simulink model "RoboBoatVU_2014_Athena"  (R2014a)
settings: Solver=FixedStepDiscrete  StartTime=0.0  StopTime=inf  FixedStep=.1  RelTol=1e-3
undefined symbols (not defined in the file): Com1, Com2, Com3, Com4, DiscIntNeverNeededParam, RGB24, standard, strel
libraries: visiontextngfix x25, dspmtrx3 x22, simulink x19, xpcseriallib x12, slrtlib x7, speedgoatlib_IO102 x6, dspstat3 x5, visionstatistics x3, dspindex x2, xpcvideousblib x2, xpcvideoutillib x2, visionmorphops x1
(part 2 of 4)

== matlab function RoboBoatVU_2014_Athena/Main FSM/Start Speed Gate/Start Speed Gate - Color/Nav Finished ==
  data: Timer input; Finished output; Timeout input; EndGPS input; Latitude input; Longitude input
function Finished = NavFinished(Timer, Timeout, EndGPS, Latitude, Longitude)

%Written by Anderson Lebbad on August 23, 2013
%Last Edited by:

%Checks the timeout and GPS location to determine if the navigation block
%is done. If either one is flagged, the finished signal is sent.


%Parse input GPS and convert angles to radians
CurLat = (floor(Latitude/100)+mod(Latitude,100)/60)*pi/180;
CurLong = (floor(Longitude/100)+mod(Longitude,100)/60)*pi/180;
DesLat = (floor(EndGPS(1)/100)+mod(EndGPS(1),100)/60)*pi/180;
DesLong = (floor(EndGPS(2)/100)+mod(EndGPS(2),100)/60)*pi/180;


%Initialize output
Finished = 0;


%Difference between lats and longs
DiffLat = DesLat - CurLat;
DiffLong = DesLong - CurLong;


%Radius of the earth in meters
R = 6378137;


%Calculate distance using the great-circle distance formula
%Formula documented here:
%   http://www.movable-type.co.uk/scripts/latlong.html
a = sin(DiffLat/2)^2+sin(DiffLong/2)^2*cos(CurLat)*cos(DesLat);
c = 2*atan2(sqrt(a), sqrt(1-a));
Distance = R*c;


%Check timeout and distance, minimum distance to pass a finished signal is
%set to 2 meters
if (Timer > Timeout) || (Distance < 2)
    Finished = 1;
end

== matlab function RoboBoatVU_2014_Athena/Parameters/Task Selector/Message Composer2 ==
  data: taskStrInit input; taskStrAdj output
function taskStrAdj = composeMessage(taskStrInit)
%Written by Anderson Lebbad on August 9, 2013
%Last Edited: Edward Zhu on June 2, 2014

%This function adjusts the length of a vector to a set value by filling
%the remaining space with 0's. This is necessary for data store objects
%that have a fixed size for the memory allocation, but a variable length
%input.

%Length of message packet
strLength = 8;

%Size of text in message
taskStrLength = size(taskStrInit,1);

%Pad end of text with zeros
taskStrAdj = [taskStrInit' zeros(1,strLength-taskStrLength)];

== matlab function RoboBoatVU_2014_Athena/Parameters/Task Selector/Message Composer5 ==
  data: taskStrInit input; taskStrAdj output
function taskStrAdj = composeMessage(taskStrInit)
%Written by Anderson Lebbad on August 9, 2013
%Last Edited: Edward Zhu on June 2, 2014

%This function adjusts the length of a vector to a set value by filling
%the remaining space with 0's. This is necessary for data store objects
%that have a fixed size for the memory allocation, but a variable length
%input.

%Length of message packet
strLength = 8;

%Size of text in message
taskStrLength = size(taskStrInit,1);

%Pad end of text with zeros
taskStrAdj = [taskStrInit' zeros(1,strLength-taskStrLength)];

== matlab function RoboBoatVU_2014_Athena/Main FSM/Start Speed Gate/Start Speed Gate - Color/Buoy Decisions/Nav Logic ==
  data: Compass input; RedBBox input; GreenBBox input; RedCentroid input; GreenCentroid input; Course input; RedDist output; GreenDist output; RPM output; DesiredHeading output; Timer input
function [RedDist, GreenDist, RPM, DesiredHeading] = NavLogic(Compass,...
    RedBBox, GreenBBox, RedCentroid, GreenCentroid, Course, Timer)

%Written by Anderson Lebbad on August 20, 2013
%Last Edited by:

%Determines the signals for driving through the buoy channel based on the
%bounding box and centroid signals from both the red and green detection
%blocks.


%Initialize Outputs
RPM = 2800;
DesiredHeading = Compass;



%% First, calculate the distance each detected polyform A-0 buoy is.

%The buoy has a fixed diameter (m), the camera has a known field of view
%(which will be converted to radians for calculations) and the size of the
%frame (in pixels) is fixed
diameter = 0.3556;
FoV = 62*pi/180;
wFrame = 640;


%The bounding box passes the width of the found buoy in pixels
wRedBox = RedBBox(3);
wGreenBox = GreenBBox(3);


%The ratio of the widths in pixels corresponds to the ratio of the withs in
%meters, and the width of the frame in meters is equal to the angle of the
%field of view (in radians) multiplied by the distance it is away from the
%buoy
RedDist = (wFrame * diameter) / (wRedBox * FoV);
GreenDist = (wFrame * diameter) / (wGreenBox * FoV);



%% Second, determine angles to buoys and offset angles for steering

%Reference angle measured from bottom center of the frame (image
%coordinates are referenced to top left corner of image, with higher x
%values being more towards the right of the image, and higher y values
%being more towards the bottom of the image)
RedX = RedCentroid(1) - 320;
RedY = 480 - RedCentroid(2);
GreenX = GreenCentroid(1) - 320;
GreenY = 480 - GreenCentroid(2);


%Return angles in degrees
RedAngle = atan(RedX / RedY) * 180 / pi;
GreenAngle = atan(GreenX / GreenY) * 180 / pi;


%Buffer for single buoy offset is the angle to twice the boat's width off of the
%center of the buoy
BoatWidth = .75;
Buffer = atan(2 * BoatWidth / RedDist) * 180 / pi;


%Red offset is to the right and green is to the left to stay within gates
RedOffset = RedAngle + Buffer;
GreenOffset = GreenAngle - Buffer;



%% Third, determine whether both buoys are located and whether or not
%navigation can treat them as a pair. 

%Check to see if a valid value was passed for the centroid for both the red
%and green blobs
if RedCentroid(1) == -1
    RedLocate = 0;
else
    RedLocate = 1;
end
if GreenCentroid(1) == -1
    GreenLocate = 0;
else
    GreenLocate = 1;
end


%if both are located and red is to the left of green, steer between the
%two. Otherwise, do appropriate one buoy navigation, or mark no buoys as
%found
if RedLocate == 1 && GreenLocate == 1
    if RedAngle < GreenAngle
        DesiredHeading = mod(Compass + (RedAngle + GreenAngle) / 2, 360);
        RPM = 4000;
    elseif Course == 'A'
        DesiredHeading = mod(Compass + RedOffset, 360);
    else
        DesiredHeading = mod(Compass + GreenOffset, 360);
    end
    buoysFound = 2;
elseif RedLocate == 1
    DesiredHeading = mod(Compass + RedOffset, 360);
    buoysFound = 1;
elseif GreenLocate == 1
    DesiredHeading = mod(Compass + GreenOffset, 360);
    buoysFound = 1;
else
    buoysFound = 0;
end


%% Fourth, search algorithm if no buoys are found. The search algorithm is
%designed to first hold the last heading for two seconds (in case lighting
%and focus caused the buoys to not be detected for a few frames), then to
%turn away from the last buoy position in the opposite direction of the
%other course by the angle of the field of view, and then towards the
%direction of the other course by the angle of the field of view. If a buoy
%is not found by the time this is done, the boat orients itself back in the
%direction that a buoy was last found, and slowly backs up.

%Set a persistent variables to track the last time a buoy was detected and
%heading it was at when it saw it. 
persistent TimeLastFound
if isempty(TimeLastFound)
    TimeLastFound = Timer;
end
persistent HeadingLastFound
if isempty(HeadingLastFound)
    HeadingLastFound = Compass;
end


%Set a variable for tracking the time since the last buoy was found
TimeNoBuoys = Timer - TimeLastFound;


%Set a variable for which way to initially turn during the search algorithm
%based on the course number
if Course == 'B'
    Turn = -FoV * 180 / pi;
else
    Turn = FoV * 180 / pi;
end

%Check to see if no buoys are found, and how long it has been to determine
%what part of the search algorithm to run
if buoysFound == 0
    RPM= 0;
    if TimeNoBuoys < 5
        DesiredHeading = HeadingLastFound;
    elseif TimeNoBuoys < 6
        DesiredHeading = mod(HeadingLastFound + Turn, 360);
    elseif TimeNoBuoys < 16
        DesiredHeading = mod(HeadingLastFound - Turn, 360);
    else
        DesiredHeading = HeadingLastFound;
        RPM = -100;
    end
else
    TimeLastFound = Timer;
    HeadingLastFound = Compass;
end

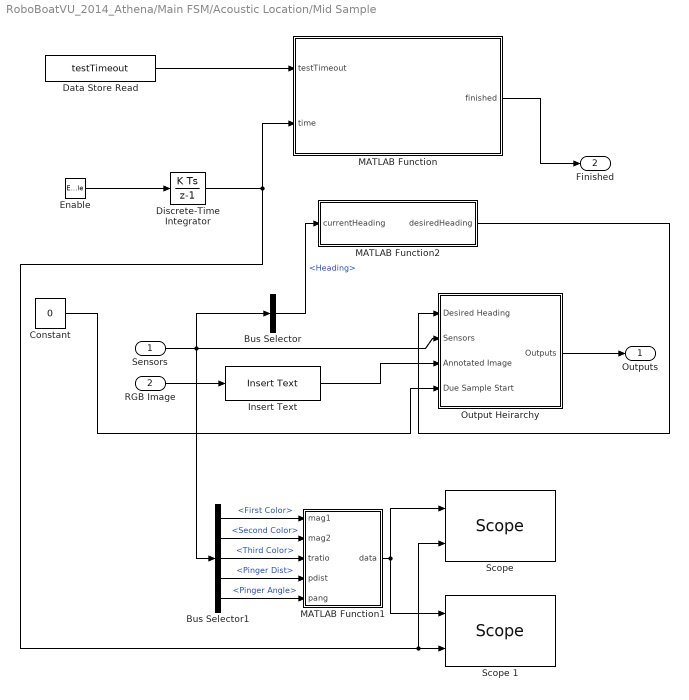
== system RoboBoatVU_2014_Athena/Main FSM/Acoustic Location/Mid Sample ==
  Sensors : Inport
  RGB Image : Inport  Port=2
  Enable : EnablePort  ShowOutputPort=on
  Bus Selector : BusSelector  OutputSignals=Serial In.Compass.Heading
  Bus Selector1 : BusSelector  OutputSignals=Serial In.Arduino Messages.First Color,Serial In.Arduino Messages.Second Color,Serial In.Arduino Messages.Third Color,Serial In.Arduino Messages.Pinger Dist,Serial In.Arduino Messages.Pinger Angle
  Constant : Constant  Value=0
  Data Store Read : DataStoreRead  DataStoreName=testTimeout
  Discrete-Time Integrator : DiscreteIntegrator  SampleTime=0.1  ICPrevOutput=DiscIntNeverNeededParam  ICPrevScaledInput=DiscIntNeverNeededParam
  Insert Text : visiontextngfix/Insert Text  inputType=Obsolete  theText='Mid Sample'  getTextLocFrom=Specify via dialog  textLoc=[1 1]  getTextColorFrom=Specify via dialog  textColor=[0 0 0]  getTextIntensityFrom=Specify via dialog  textIntensity=0  getTextOpacityFrom=Specify via dialog  textOpacity=1.0  dummyVar2=0  dummyVar3=0  dummyVar4=0  imagePorts=One multidimensional signal  isInputTransposed=off  fontFace=LucidaSansRegular  dummyVar1=0  blockFontSize=12  antiAliased=on
  MATLAB Function : MATLAB Function  TreatAsAtomicUnit=on
  MATLAB Function1 : MATLAB Function  TreatAsAtomicUnit=on
  MATLAB Function2 : MATLAB Function  TreatAsAtomicUnit=on
  Output Heirarchy : Subsystem
  "Scope " : slrtlib/Displays and Logging/Scope   scopeno=2  scopetype=File  autostart=on  viewmode=Graphical redraw  formatstr='%15.6f'  grid=on  ylimits=[0,0]  nosamples=100  noprepostsamples=0  interleave=1  triggermode=Signal triggering  triggersignal=1  trigsignalfromport=on  triggerlevel=1  triggerslope=Either  triggerscope=1  triggersample=0  filename=msample2.dat  mode=Lazy  writesize=512  autorestart=off  dynamicfilemode=off  maxwritefilesize=512*1024^2
  Scope 1 : slrtlib/Displays and Logging/Scope   scopeno=3  scopetype=Host  autostart=on  viewmode=Graphical redraw  formatstr='%15.6f'  grid=on  ylimits=[0,0]  nosamples=100  noprepostsamples=0  interleave=1  triggermode=Signal triggering  triggersignal=1  trigsignalfromport=on  triggerlevel=1  triggerslope=Either  triggerscope=1  triggersample=0  filename=msample1.dat  mode=Lazy  writesize=512  autorestart=off  dynamicfilemode=off  maxwritefilesize=512*1024^2
  Outputs : Outport
  Finished : Outport  Port=2
  wires:
  RGB Image/1 -> Insert Text/1
  Insert Text/1 -> Output Heirarchy/3(Annotated Image)
  Bus Selector/1 -> MATLAB Function2/1(currentHeading)  "<Heading>"
  Output Heirarchy/1(Outputs) -> Outputs/1
  Data Store Read/1 -> MATLAB Function/1(testTimeout)
  MATLAB Function/1(finished) -> Finished/1
  Enable/1 -> Discrete-Time Integrator/1
  Sensors/1 -> Bus Selector1/1, Bus Selector/1, Output Heirarchy/2(Sensors)
  Bus Selector1/5 -> MATLAB Function1/5(pang)  "<Pinger Angle>"
  Bus Selector1/2 -> MATLAB Function1/2(mag2)  "<Second Color>"
  Bus Selector1/1 -> MATLAB Function1/1(mag1)  "<First Color>"
  Bus Selector1/3 -> MATLAB Function1/3(tratio)  "<Third Color>"
  Bus Selector1/4 -> MATLAB Function1/4(pdist)  "<Pinger Dist>"
  MATLAB Function1/1(data) -> "Scope "/1, Scope 1/1
  Constant/1 -> Output Heirarchy/4(Due Sample Start)
  Discrete-Time Integrator/1 -> Scope 1/2, "Scope "/2, MATLAB Function/2(time)
  MATLAB Function2/1(desiredHeading) -> Output Heirarchy/1(Desired Heading)

== system RoboBoatVU_2014_Athena/Main FSM/Acoustic Location/Right Sample ==
  Sensors : Inport
  RGB Image : Inport  Port=2
  Enable : EnablePort  ShowOutputPort=on
  Bus Selector : BusSelector  OutputSignals=Serial In.Compass.Heading
  Bus Selector1 : BusSelector  OutputSignals=Serial In.Arduino Messages.First Color,Serial In.Arduino Messages.Second Color,Serial In.Arduino Messages.Third Color,Serial In.Arduino Messages.Pinger Dist,Serial In.Arduino Messages.Pinger Angle
  Constant : Constant  Value=0
  Data Store Read : DataStoreRead  DataStoreName=testTimeout
  Discrete-Time Integrator : DiscreteIntegrator  SampleTime=0.1  ICPrevOutput=DiscIntNeverNeededParam  ICPrevScaledInput=DiscIntNeverNeededParam
  Insert Text : visiontextngfix/Insert Text  inputType=Obsolete  theText='Right Sample'  getTextLocFrom=Specify via dialog  textLoc=[1 1]  getTextColorFrom=Specify via dialog  textColor=[0 0 0]  getTextIntensityFrom=Specify via dialog  textIntensity=0  getTextOpacityFrom=Specify via dialog  textOpacity=1.0  dummyVar2=0  dummyVar3=0  dummyVar4=0  imagePorts=One multidimensional signal  isInputTransposed=off  fontFace=LucidaSansRegular  dummyVar1=0  blockFontSize=12  antiAliased=on
  MATLAB Function : MATLAB Function  TreatAsAtomicUnit=on
  MATLAB Function1 : MATLAB Function  TreatAsAtomicUnit=on
  MATLAB Function2 : MATLAB Function  TreatAsAtomicUnit=on
  Output Heirarchy1 : Subsystem
  "Scope " : slrtlib/Displays and Logging/Scope   scopeno=6  scopetype=File  autostart=on  viewmode=Graphical redraw  formatstr='%15.6f'  grid=on  ylimits=[0,0]  nosamples=100  noprepostsamples=0  interleave=1  triggermode=Signal triggering  triggersignal=1  trigsignalfromport=on  triggerlevel=1  triggerslope=Either  triggerscope=1  triggersample=0  filename=rsample3.dat  mode=Lazy  writesize=512  autorestart=off  dynamicfilemode=off  maxwritefilesize=512*1024^2
  Scope 1 : slrtlib/Displays and Logging/Scope   scopeno=7  scopetype=Host  autostart=on  viewmode=Graphical redraw  formatstr='%15.6f'  grid=on  ylimits=[0,0]  nosamples=100  noprepostsamples=0  interleave=1  triggermode=Signal triggering  triggersignal=1  trigsignalfromport=on  triggerlevel=1  triggerslope=Either  triggerscope=1  triggersample=0  filename=msample1.dat  mode=Lazy  writesize=512  autorestart=off  dynamicfilemode=off  maxwritefilesize=512*1024^2
  Outputs : Outport
  wires:
  RGB Image/1 -> Insert Text/1
  Insert Text/1 -> Output Heirarchy1/4(Annotated Image)
  Bus Selector/1 -> MATLAB Function2/1(currentHeading)  "<Heading>"
  Output Heirarchy1/1(Outputs) -> Outputs/1
  Data Store Read/1 -> MATLAB Function/1(testTimeout)
  Enable/1 -> Discrete-Time Integrator/1
  MATLAB Function/1(finished) -> Output Heirarchy1/1(Finished)
  Sensors/1 -> Bus Selector/1, Bus Selector1/1, Output Heirarchy1/3(Sensors)
  Bus Selector1/5 -> MATLAB Function1/5(pang)  "<Pinger Angle>"
  Bus Selector1/2 -> MATLAB Function1/2(mag2)  "<Second Color>"
  Bus Selector1/1 -> MATLAB Function1/1(mag1)  "<First Color>"
  Bus Selector1/3 -> MATLAB Function1/3(tratio)  "<Third Color>"
  Bus Selector1/4 -> MATLAB Function1/4(pdist)  "<Pinger Dist>"
  MATLAB Function1/1(data) -> "Scope "/1, Scope 1/1
  Constant/1 -> Output Heirarchy1/5(Due Sample Start)
  Discrete-Time Integrator/1 -> Scope 1/2, "Scope "/2, MATLAB Function/2(time)
  MATLAB Function2/1(desiredHeading) -> Output Heirarchy1/2(Desired Heading)

== system RoboBoatVU_2014_Athena/Main FSM/Acoustic Location/Right Turn ==
  Sensors : Inport
  RGB Image : Inport  Port=2
  Enable : EnablePort
  Bus Selector : BusSelector  OutputSignals=Serial In.Compass.Heading
  Constant : Constant  Commented=on
  Insert Text : visiontextngfix/Insert Text  inputType=Obsolete  theText='Right Turn'  getTextLocFrom=Specify via dialog  textLoc=[1 1]  getTextColorFrom=Specify via dialog  textColor=[0 0 0]  getTextIntensityFrom=Specify via dialog  textIntensity=0  getTextOpacityFrom=Specify via dialog  textOpacity=1.0  dummyVar2=0  dummyVar3=0  dummyVar4=0  imagePorts=One multidimensional signal  isInputTransposed=off  fontFace=LucidaSansRegular  dummyVar1=0  blockFontSize=12  antiAliased=on
  Output Heirarchy : Subsystem
  Right Turn : MATLAB Function  TreatAsAtomicUnit=on
  Outputs : Outport
  Finished : Outport  Port=2
  wires:
  Sensors/1 -> Output Heirarchy/2(Sensors), Bus Selector/1
  Bus Selector/1 -> Right Turn/1(currentHeading)  "<Heading>"
  Right Turn/1(desiredHeading) -> Output Heirarchy/1(Desired Heading)
  RGB Image/1 -> Insert Text/1
  Insert Text/1 -> Output Heirarchy/3(Annotated Image)
  Output Heirarchy/1(Outputs) -> Outputs/1
  Right Turn/2(finished) -> Finished/1

== system RoboBoatVU_2014_Athena/Main FSM/Color Sequence Detection/Output Heirarchy1 ==
  Arduino Ready : Inport
  Annotated Image : Inport  Port=2
  Desired Heading : Inport  Port=3
  Sensors : Inport  Port=4
  Bus Creator : BusCreator  Inputs=3
  Bus Creator1 : BusCreator  Inputs=2
  Bus Creator2 : BusCreator  Inputs=3
  Bus Creator3 : BusCreator  Inputs=2
  Bus Creator4 : BusCreator  Inputs=2
  Due Sample Start : Constant  Value=0
  Finished : Constant  Value=0
  RPM Desired : Constant  Value=0
  Uno Power : Constant
  Outputs : Outport
  wires:
  RPM Desired/1 -> Bus Creator/1  "RPM"
  Bus Creator/1 -> Bus Creator1/1  "Control Signals"
  Bus Creator2/1 -> Bus Creator/3  "Arduino Signals"
  Uno Power/1 -> Bus Creator2/2  "Uno Power"
  Desired Heading/1 -> Bus Creator/2  "Desired Heading"
  Bus Creator1/1 -> Bus Creator4/1  "Outputs"
  Annotated Image/1 -> Bus Creator1/2  "Annotated Image"
  Sensors/1 -> Bus Creator4/2  "Sensors"
  Bus Creator4/1 -> Bus Creator3/1  "Output Signals"
  Arduino Ready/1 -> Bus Creator2/1  "Ready to Read"
  Due Sample Start/1 -> Bus Creator2/3  "Due Sample Start"
  Bus Creator3/1 -> Outputs/1
  Finished/1 -> Bus Creator3/2  "Task Finished"

== system RoboBoatVU_2014_Athena/Main FSM/Docking/Blob Analysis ==
  RGB Image : Inport
  Blob Analysis : visionstatistics/Blob Analysis  Tag=vipblks_row_conv  area=off  centroid=off  bBox=on  majorAxis=off  minorAxis=off  angle=off  eccentricity=off  equivDiameterSq=off  extent=off  perimeter=off  maxBlobs=10  warnIfNumBlobsExceeded=on  isCount=off  useMinArea=on  minArea=700  useMaxArea=off  maxArea=intmax('uint32')  excludeBorderBlob=on  outDT=double  isOutVarDim=off  isFill=on  fillValues=-1  conn=8  isLabel=on  outputMode=Binary point scaling  outputWordLength=32  outputFracLength=16  firstCoeffMode=Binary point scaling  firstCoeffWordLength=16  firstCoeffFracLength=14  secondCoeffMode=Binary point scaling  secondCoeffWordLength=32  secondCoeffFracLength=16  accumMode=Binary point scaling  accumWordLength=32  accumFracLength=0  prodOutputMode=Binary point scaling  prodOutputWordLength=32  prodOutputFracLength=16  roundingMode=Floor  overflowMode=off
  Closing : visionmorphops/Closing  nhoodsrc=Specify via dialog  strel=strel('disk',1,4)
  Compare To Constant : simulink/Logic and Bit Operations/Compare To Constant  relop=<=  const=100  OutDataTypeStr=boolean
  S-Function : S-Function  FunctionName=rgbtohsv_int_sfun  EnableBusSupport=off
  Selector : Selector  NumberOfDimensions=3  InputPortWidth=3  IndexOptions=Select all,Select all,Index vector (dialog)  Indices=[1 3],1,3  OutputSizes=1,1,1
  Submatrix : dspmtrx3/Submatrix  RowSpan=Range of rows  RowStartMode=First  RowStartIndex=1  RowEndMode=Index  RowEndIndex=240  ColSpan=Range of columns  ColStartMode=First  ColStartIndex=128  ColEndMode=Last  ColEndIndex=1
  "BBox " : Outport
  Label : Outport  Port=2
  V mask : Outport  Port=3
  wires:
  RGB Image/1 -> S-Function/1
  S-Function/1 -> Selector/1
  Selector/1 -> Submatrix/1
  Submatrix/1 -> Compare To Constant/1
  Blob Analysis/1 -> "BBox "/1
  Blob Analysis/2 -> Label/1
  Compare To Constant/1 -> Closing/1
  Closing/1 -> V mask/1, Blob Analysis/1

== system RoboBoatVU_2014_Athena/Main FSM/Docking/Detection ==
  Parameters : Inport
  BBox In : Inport  Port=2
  Label : Inport  Port=3
  V Mask : Inport  Port=4
  Bus Selector2 : BusSelector  OutputSignals=Templates.Cruciform,Templates.Circle,Templates.Triangle,White Pix Count,Threshold
  Detection : MATLAB Function  TreatAsAtomicUnit=on
  Sort and Filter for Best Three : Subsystem
  BBox Out : Outport
  wires:
  Bus Selector2/1 -> Detection/1(cruciform)  "<Cruciform>"
  Bus Selector2/2 -> Detection/2(circle)  "<Circle>"
  Bus Selector2/3 -> Detection/3(triangle)  "<Triangle>"
  Bus Selector2/4 -> Detection/4(whitePixCount)  "<White Pix Count>"
  Bus Selector2/5 -> Detection/5(threshold)  "<Threshold>"
  Detection/1(bbox_out) -> Sort and Filter for Best Three/1(BBox in)
  Detection/2(rtnRatioDiff) -> Sort and Filter for Best Three/2(Idx)
  Parameters/1 -> Bus Selector2/1
  Sort and Filter for Best Three/1(BBox out) -> BBox Out/1
  V Mask/1 -> Detection/6(V_mask)
  BBox In/1 -> Detection/7(bbox_in)
  Label/1 -> Detection/8(label)

== system RoboBoatVU_2014_Athena/Main FSM/Docking/Output Heirarchy2 ==
  Annotated Image : Inport
  Desired Heading : Inport  Port=2
  Sensors : Inport  Port=3
  Bus Creator : BusCreator  Inputs=3
  Bus Creator1 : BusCreator  Inputs=2
  Bus Creator2 : BusCreator  Inputs=3
  Bus Creator3 : BusCreator  Inputs=2
  Bus Creator4 : BusCreator  Inputs=2
  Due Sample Start : Constant  Value=0
  Finished : Constant  Value=0
  RPM Desired : Constant  Value=0
  Ready to Read : Constant  Value=0
  Uno Power : Constant  Value=0
  Outputs : Outport
  wires:
  RPM Desired/1 -> Bus Creator/1  "RPM"
  Bus Creator/1 -> Bus Creator1/1  "Control Signals"
  Bus Creator2/1 -> Bus Creator/3  "Arduino Signals"
  Uno Power/1 -> Bus Creator2/2  "Uno Power"
  Desired Heading/1 -> Bus Creator/2  "Desired Heading"
  Bus Creator1/1 -> Bus Creator4/1  "Outputs"
  Annotated Image/1 -> Bus Creator1/2  "Annotated Image"
  Sensors/1 -> Bus Creator4/2  "Sensors"
  Bus Creator4/1 -> Bus Creator3/1  "Output Signals"
  Ready to Read/1 -> Bus Creator2/1  "Ready to Read"
  Due Sample Start/1 -> Bus Creator2/3  "Due Sample Start"
  Bus Creator3/1 -> Outputs/1
  Finished/1 -> Bus Creator3/2  "Task Finished"

== system RoboBoatVU_2014_Athena/Main FSM/Docking/Parameters ==
  note: Target template
      | 1 - cruciform
      | 2 - circle
      | 3 - triangle
  Bus Creator : BusCreator
  Ratio Difference Threshold : Constant  Value=0.7
  Target Template : Constant  Value=2
  Templates : Subsystem
  White Pixel Count : Constant  Value="[144\t64\t180]"
  Parameters : Outport
  wires:
  Templates/1(Templates) -> Bus Creator/2  "Templates"
  White Pixel Count/1 -> Bus Creator/3  "White Pix Count"
  Bus Creator/1 -> Parameters/1  "Parameters"
  Ratio Difference Threshold/1 -> Bus Creator/4  "Threshold"
  Target Template/1 -> Bus Creator/1  "Target Template"

== system RoboBoatVU_2014_Athena/Main FSM/Docking/Recognition ==
  Parameters : Inport
  BBox In : Inport  Port=2
  V Mask : Inport  Port=3
  Bus Selector3 : BusSelector  OutputSignals=Target Template,Templates.Cruciform,Templates.Circle,Templates.Triangle,White Pix Count,Threshold
  Recognition : MATLAB Function  TreatAsAtomicUnit=on
  Sort and Filter for Best One : Subsystem
  BBox Out : Outport
  wires:
  Bus Selector3/1 -> Recognition/1(targetTemp)  "<Target Template>"
  Bus Selector3/2 -> Recognition/2(cruciform)  "<Cruciform>"
  Bus Selector3/3 -> Recognition/3(circle)  "<Circle>"
  Bus Selector3/4 -> Recognition/4(triangle)  "<Triangle>"
  Bus Selector3/5 -> Recognition/5(whitePixCount)  "<White Pix Count>"
  Bus Selector3/6 -> Recognition/6(threshold)  "<Threshold>"
  Recognition/1(bbox_out) -> Sort and Filter for Best One/1(BBox in)
  Parameters/1 -> Bus Selector3/1
  Sort and Filter for Best One/1(BBox out) -> BBox Out/1
  Recognition/2(returnRatioDiff) -> Sort and Filter for Best One/2(Idx)
  V Mask/1 -> Recognition/7(V_mask)
  BBox In/1 -> Recognition/8(bbox_in)

== system RoboBoatVU_2014_Athena/Main FSM/Docking/Video Annotation ==
  RGB Image : Inport
  BBox Recognition : Inport  Port=2
  BBox Detect : Inport  Port=3
  Bay Number : Inport  Port=4
  Draw Shapes : visiontextngfix/Draw Shapes  shape=Rectangles  fill=on  lineWidth=1  fillClrSource=Specify via dialog  display=User-specified value  intensity=200  color=[0 0 100]  opacity=0.6  viewport=Entire image  antialiasing=off  inType=Obsolete  imagePorts=One multidimensional signal  prodOutputMode=Binary point scaling  prodOutputWordLength=32  prodOutputFracLength=14  memoryMode=Specify word length  memoryWordLength=16  memoryFracLength=14  roundingMode=Floor  overflowMode=off
  Draw Shapes1 : visiontextngfix/Draw Shapes  shape=Rectangles  fill=on  lineWidth=1  fillClrSource=Specify via dialog  display=User-specified value  intensity=200  color=[100 0 0]  opacity=0.6  viewport=Entire image  antialiasing=off  inType=Obsolete  imagePorts=One multidimensional signal  prodOutputMode=Binary point scaling  prodOutputWordLength=32  prodOutputFracLength=14  memoryMode=Specify word length  memoryWordLength=16  memoryFracLength=14  roundingMode=Floor  overflowMode=off
  Insert Text : visiontextngfix/Insert Text  inputType=Obsolete  theText='Target Bay: %i'  getTextLocFrom=Specify via dialog  textLoc=[1 1]  getTextColorFrom=Specify via dialog  textColor=[0 0 0]  getTextIntensityFrom=Specify via dialog  textIntensity=0  getTextOpacityFrom=Specify via dialog  textOpacity=1.0  dummyVar2=0  dummyVar3=0  dummyVar4=0  imagePorts=One multidimensional signal  isInputTransposed=off  fontFace=LucidaSansRegular  dummyVar1=0  blockFontSize=12  antiAliased=on
  x shift : MATLAB Function  Commented=through  TreatAsAtomicUnit=on
  Out1 : Outport
  wires:
  BBox Detect/1 -> x shift/1(bbox_in)
  RGB Image/1 -> Draw Shapes/1
  x shift/1(bbox_out) -> Draw Shapes/2
  Draw Shapes/1 -> Draw Shapes1/1
  BBox Recognition/1 -> Draw Shapes1/2
  Draw Shapes1/1 -> Insert Text/1
  Bay Number/1 -> Insert Text/2
  Insert Text/1 -> Out1/1

== system RoboBoatVU_2014_Athena/Main FSM/Initialization/Output Heirarchy ==
  Annotated Image : Inport
  Desired Heading : Inport  Port=2
  Sensors : Inport  Port=3
  Bus Creator : BusCreator  Inputs=3
  Bus Creator1 : BusCreator  Inputs=2
  Bus Creator2 : BusCreator  Inputs=3
  Bus Creator3 : BusCreator  Inputs=2
  Bus Creator4 : BusCreator  Inputs=2
  Due Sample Start : Constant  Value=0
  Finished : Constant  Value=0
  RPM Desired : Constant  Value=0
  Ready to Read : Constant  Value=0
  Uno Power : Constant  Value=0
  Outputs : Outport
  wires:
  RPM Desired/1 -> Bus Creator/1  "RPM"
  Bus Creator/1 -> Bus Creator1/1  "Control Signals"
  Bus Creator2/1 -> Bus Creator/3  "Arduino Signals"
  Uno Power/1 -> Bus Creator2/2  "Uno Power"
  Desired Heading/1 -> Bus Creator/2  "Desired Heading"
  Bus Creator1/1 -> Bus Creator4/1  "Outputs"
  Annotated Image/1 -> Bus Creator1/2  "Annotated Image"
  Sensors/1 -> Bus Creator4/2  "Sensors"
  Bus Creator4/1 -> Bus Creator3/1  "Output Signals"
  Ready to Read/1 -> Bus Creator2/1  "Ready to Read"
  Due Sample Start/1 -> Bus Creator2/3  "Due Sample Start"
  Bus Creator3/1 -> Outputs/1
  Finished/1 -> Bus Creator3/2  "Task Finished"

== system RoboBoatVU_2014_Athena/Main FSM/Obstacle Navigation/Output Heirarchy1 ==
  Desired Heading : Inport
  Sensors : Inport  Port=2
  Annotated Image : Inport  Port=3
  Bus Creator : BusCreator  Inputs=3
  Bus Creator1 : BusCreator  Inputs=2
  Bus Creator2 : BusCreator  Inputs=3
  Bus Creator3 : BusCreator  Inputs=2
  Bus Creator4 : BusCreator  Inputs=2
  Due Sample Start : Constant  Value=0
  Finished : Constant  Value=0
  RPM Desired : Constant  Value=0
  Ready to Read : Constant  Value=0
  Uno Power : Constant  Value=0
  Outputs : Outport
  wires:
  RPM Desired/1 -> Bus Creator/1  "RPM"
  Bus Creator/1 -> Bus Creator1/1  "Control Signals"
  Bus Creator2/1 -> Bus Creator/3  "Arduino Signals"
  Uno Power/1 -> Bus Creator2/2  "Uno Power"
  Desired Heading/1 -> Bus Creator/2  "Desired Heading"
  Bus Creator1/1 -> Bus Creator4/1  "Outputs"
  Annotated Image/1 -> Bus Creator1/2  "Annotated Image"
  Sensors/1 -> Bus Creator4/2  "Sensors"
  Bus Creator4/1 -> Bus Creator3/1  "Output Signals"
  Ready to Read/1 -> Bus Creator2/1  "Ready to Read"
  Due Sample Start/1 -> Bus Creator2/3  "Due Sample Start"
  Bus Creator3/1 -> Outputs/1
  Finished/1 -> Bus Creator3/2  "Task Finished"

== system RoboBoatVU_2014_Athena/Main FSM/RCHold/Output Heirarchy1 ==
  Annotated Image : Inport
  Desired Heading : Inport  Port=2
  Sensors : Inport  Port=3
  Bus Creator : BusCreator  Inputs=3
  Bus Creator1 : BusCreator  Inputs=2
  Bus Creator2 : BusCreator  Inputs=3
  Bus Creator3 : BusCreator  Inputs=2
  Bus Creator4 : BusCreator  Inputs=2
  Due Sample Start : Constant  Value=0
  Finished : Constant  Value=0
  RPM Desired : Constant  Value=0
  Ready to Read : Constant  Value=0
  Uno Power : Constant  Value=0
  Outputs : Outport
  wires:
  RPM Desired/1 -> Bus Creator/1  "RPM"
  Bus Creator/1 -> Bus Creator1/1  "Control Signals"
  Bus Creator2/1 -> Bus Creator/3  "Arduino Signals"
  Uno Power/1 -> Bus Creator2/2  "Uno Power"
  Desired Heading/1 -> Bus Creator/2  "Desired Heading"
  Bus Creator1/1 -> Bus Creator4/1  "Outputs"
  Annotated Image/1 -> Bus Creator1/2  "Annotated Image"
  Sensors/1 -> Bus Creator4/2  "Sensors"
  Bus Creator4/1 -> Bus Creator3/1  "Output Signals"
  Ready to Read/1 -> Bus Creator2/1  "Ready to Read"
  Due Sample Start/1 -> Bus Creator2/3  "Due Sample Start"
  Bus Creator3/1 -> Outputs/1
  Finished/1 -> Bus Creator3/2  "Task Finished"

== system RoboBoatVU_2014_Athena/Main FSM/Return to Start/GPS: Center ==
  Sensors : Inport
  RGB image : Inport  Port=2
  Enable : EnablePort
  Approach : Subsystem  TreatAsAtomicUnit=on
  GPS Enabler : MATLAB Function  TreatAsAtomicUnit=on
  GPS Selector : MultiPortSwitch  Inputs=2
  Orient : Subsystem  TreatAsAtomicUnit=on
  Output Reassign : Subsystem
  Unit Delay : UnitDelay  SampleTime=-1
  Outputs : Outport
  Finished : Outport  Port=2
  wires:
  Sensors/1 -> Approach/1(Sensors), Orient/1(Sensors)
  GPS Enabler/2(OrientEnable) -> Orient/Enable
  GPS Enabler/3(ApproachEnable) -> Approach/Enable
  Orient/2(Finished) -> Unit Delay/1
  Orient/1(Outputs) -> GPS Selector/2
  Approach/1(Outputs) -> GPS Selector/3
  GPS Enabler/1(GPSMode) -> GPS Selector/1
  Unit Delay/1 -> GPS Enabler/1(Finished)
  GPS Selector/1 -> Output Reassign/1(Outputs in)
  Output Reassign/1(Outputs) -> Outputs/1
  Output Reassign/2(Finished) -> Finished/1
  RGB image/1 -> Approach/2(RGB image), Orient/2(RGB image)

== system RoboBoatVU_2014_Athena/Main FSM/Start Speed Gate/Start Speed Gate - Color ==
  Sensors : Inport
  RGB Image : Inport  Port=2
  Enable : EnablePort  ShowOutputPort=on
  Buoy Decisions : Subsystem
  Bus Selector : BusSelector  OutputSignals=Serial In.GPS.latitude,Serial In.GPS.longitude
  Nav Finished : MATLAB Function  TreatAsAtomicUnit=on
  Output Heirarchy : Subsystem
  Read : DataStoreRead  DataStoreName=ssGateGPS
  Read1 : DataStoreRead  DataStoreName=ssGateTimeout
  Start Speed Gate Detection : Subsystem
  Timer : DiscreteIntegrator  SampleTime=-1  ICPrevOutput=DiscIntNeverNeededParam  ICPrevScaledInput=DiscIntNeverNeededParam
  Outputs : Outport
  wires:
  RGB Image/1 -> Buoy Decisions/2(RGB image), Start Speed Gate Detection/1(RGB)
  Sensors/1 -> Bus Selector/1, Output Heirarchy/1(Sensors), Buoy Decisions/1(Sensors)  "Sensors"
  Start Speed Gate Detection/1(Red + Green) -> Buoy Decisions/3(Red + Green)
  Enable/1 -> Timer/1
  Timer/1 -> Nav Finished/1(Timer), Buoy Decisions/4(Timer)
  Read1/1 -> Nav Finished/2(Timeout)
  Read/1 -> Nav Finished/3(EndGPS)
  Bus Selector/2 -> Nav Finished/5(Longitude)  "<longitude>"
  Bus Selector/1 -> Nav Finished/4(Latitude)  "<latitude>"
  Nav Finished/1(Finished) -> Output Heirarchy/5(Finished)
  Buoy Decisions/2(RPM) -> Output Heirarchy/3(RPM)
  Buoy Decisions/1(Annotated Image) -> Output Heirarchy/2(Annotated Image)
  Buoy Decisions/3(Desired Heading) -> Output Heirarchy/4(Desired Heading)
  Output Heirarchy/1(Outputs) -> Outputs/1

== system RoboBoatVU_2014_Athena/Main FSM/Start Speed Gate/Start Speed Gate - LIDAR ==
  Sensors : Inport
  RGB Image : Inport  Port=2
  Enable : EnablePort
  Output Heirarchy : Subsystem
  Output : Outport
  wires:
  Output Heirarchy/1(Outputs) -> Output/1

== system RoboBoatVU_2014_Athena/Main FSM/Termination/Output Heirarchy1 ==
  Annotated Image : Inport
  Desired Heading : Inport  Port=2
  Sensors : Inport  Port=3
  Bus Creator : BusCreator  Inputs=3
  Bus Creator1 : BusCreator  Inputs=2
  Bus Creator2 : BusCreator  Inputs=3
  Bus Creator3 : BusCreator  Inputs=2
  Bus Creator4 : BusCreator  Inputs=2
  Due Sample Start : Constant  Value=0
  Finished : Constant  Value=0
  RPM Desired : Constant  Value=0
  Ready to Read : Constant  Value=0
  Uno Power : Constant  Value=0
  Outputs : Outport
  wires:
  RPM Desired/1 -> Bus Creator/1  "RPM"
  Bus Creator/1 -> Bus Creator1/1  "Control Signals"
  Bus Creator2/1 -> Bus Creator/3  "Arduino Signals"
  Uno Power/1 -> Bus Creator2/2  "Uno Power"
  Desired Heading/1 -> Bus Creator/2  "Desired Heading"
  Bus Creator1/1 -> Bus Creator4/1  "Outputs"
  Annotated Image/1 -> Bus Creator1/2  "Annotated Image"
  Sensors/1 -> Bus Creator4/2  "Sensors"
  Bus Creator4/1 -> Bus Creator3/1  "Output Signals"
  Ready to Read/1 -> Bus Creator2/1  "Ready to Read"
  Due Sample Start/1 -> Bus Creator2/3  "Due Sample Start"
  Bus Creator3/1 -> Outputs/1
  Finished/1 -> Bus Creator3/2  "Task Finished"

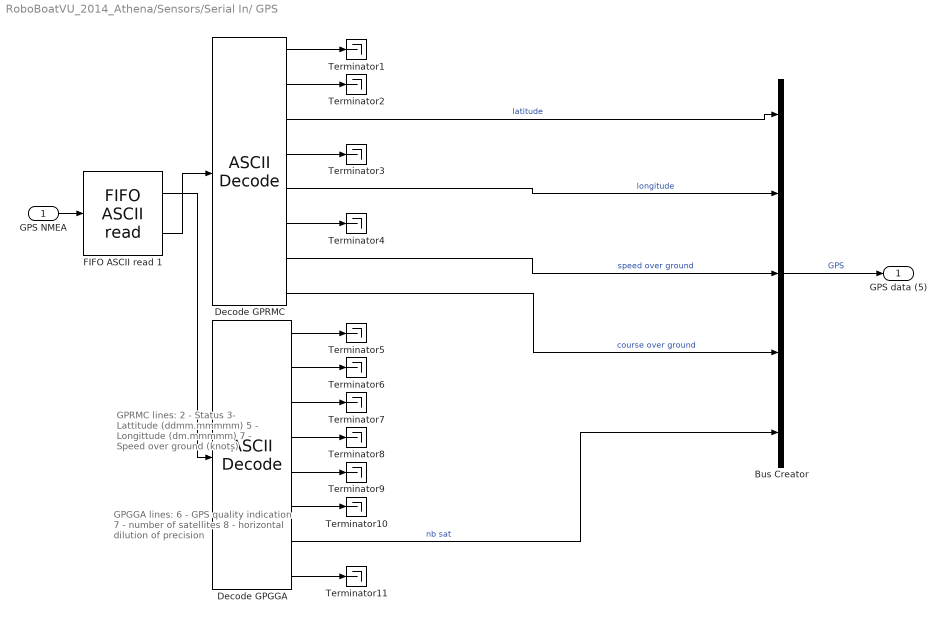
== system RoboBoatVU_2014_Athena/Sensors/Serial In/ GPS ==
  note: GPGGA lines:
      | 6 - GPS quality indication
      | 7 - number of satellites
      | 8 - horizontal dilution of precision
  note: GPRMC lines:
      | 2 - Status
      | 3- Lattitude (ddmm.mmmmm)
      | 5 - Longittude (dm.mmmmm)
      | 7 - Speed over ground (knots)
  GPS NMEA : Inport
  Bus Creator : BusCreator  Inputs=5
  Decode GPGGA : xpcseriallib/ASCII Decode   format=$GPGGA,%d,%f,%c%f,%c%f,%f,%f  nvars=8  vartypes={ }
  Decode GPRMC : xpcseriallib/ASCII Decode   format=$GPRMC,%f,%c%f,%c%f,%c%f,%f  nvars=8  vartypes={ }
  FIFO ASCII read 1 : xpcseriallib/FIFO ASCII read   header={'$GPGGA','$GPRMC'}  term=[13 10]  hold=Zero output if no new data  enable=off  maxsize=1024  outputtype=8 bit uint null terminated  sampletime=-1
  Terminator{1..11} (11 alike) : Terminator
  GPS data (5) : Outport
  wires:
  Decode GPRMC/1 -> Terminator1/1
  Decode GPRMC/7 -> Bus Creator/3  "speed over ground"
  Decode GPRMC/5 -> Bus Creator/2  "longitude"
  Decode GPRMC/3 -> Bus Creator/1  "latitude"
  GPS NMEA/1 -> FIFO ASCII read 1/1
  FIFO ASCII read 1/1 -> Decode GPGGA/1
  FIFO ASCII read 1/2 -> Decode GPRMC/1
  Decode GPRMC/8 -> Bus Creator/4  "course over ground"
  Decode GPGGA/7 -> Bus Creator/5  "nb sat"
  Decode GPRMC/2 -> Terminator2/1
  Decode GPRMC/4 -> Terminator3/1
  Decode GPRMC/6 -> Terminator4/1
  Decode GPGGA/1 -> Terminator5/1
  Decode GPGGA/2 -> Terminator6/1
  Decode GPGGA/3 -> Terminator7/1
  Decode GPGGA/4 -> Terminator8/1
  Decode GPGGA/5 -> Terminator9/1
  Decode GPGGA/6 -> Terminator10/1
  Decode GPGGA/8 -> Terminator11/1
  Bus Creator/1 -> GPS data (5)/1  "GPS"

== system RoboBoatVU_2014_Athena/Sensors/Serial In/Arduino Due ==
  Arduino Due In : Inport
  ASCII Decode 1 : xpcseriallib/ASCII Decode   format=FC:%04d,SC:%04d,TC:%04d,PD:%04d,PA:%04d\r\n  nvars=5  vartypes={'double'}
  Bus Creator : BusCreator  Inputs=5
  "FIFO ASCII read " : xpcseriallib/FIFO ASCII read   header={'FC:'}  term=[13 10]  hold=Zero output if no new data  enable=off  maxsize=1024  outputtype=8 bit uint null terminated  sampletime=0.1
  Arduino Due Out : Outport
  wires:
  "FIFO ASCII read "/1 -> ASCII Decode 1/1
  Arduino Due In/1 -> "FIFO ASCII read "/1
  ASCII Decode 1/1 -> Bus Creator/1  "First Color"
  ASCII Decode 1/2 -> Bus Creator/2  "Second Color"
  ASCII Decode 1/3 -> Bus Creator/3  "Third Color"
  ASCII Decode 1/4 -> Bus Creator/4  "Pinger Dist"
  ASCII Decode 1/5 -> Bus Creator/5  "Pinger Angle"
  Bus Creator/1 -> Arduino Due Out/1  "Arduino Messages"

== system RoboBoatVU_2014_Athena/Sensors/Serial In/Decode Compass ==
  note: Status Field can be one of the following:
      | L = low alarm
      | M= low warning
      | N = Normal
      | O = High Warning
      | P = High Alarm
      | C = Tuning analog circuit
  note: Compas NMEA- Raw data from the Compass
  Compass NMEA : Inport
  "ASCII Decode " : xpcseriallib/ASCII Decode   format=$PTNTHPR,%f,%c%f,%c%f,%c  nvars=7  vartypes={ }
  Bus Creator : BusCreator  Inputs=3
  Correct Heading Angle Magnetic to True North : Subsystem
  "FIFO ASCII read " : xpcseriallib/FIFO ASCII read   header={'$PTNTHPR'}  term=[13 10]  hold=Zero output if no new data  enable=off  maxsize=64  outputtype=8 bit uint null terminated  sampletime=-1
  Terminator{,1..3} (4 alike) : Terminator
  Compass data (3) : Outport
  wires:
  "FIFO ASCII read "/1 -> "ASCII Decode "/1
  Compass NMEA/1 -> "FIFO ASCII read "/1
  "ASCII Decode "/2 -> Terminator/1
  "ASCII Decode "/4 -> Terminator1/1
  "ASCII Decode "/6 -> Terminator2/1
  "ASCII Decode "/7 -> Terminator3/1
  Bus Creator/1 -> Compass data (3)/1  "Compass"
  "ASCII Decode "/3 -> Bus Creator/2  "Pitch"
  "ASCII Decode "/5 -> Bus Creator/3  "Roll"
  "ASCII Decode "/1 -> Correct Heading Angle Magnetic to True North/1(Heading Mag)  "Heading"
  Correct Heading Angle Magnetic to True North/1(Heading True) -> Bus Creator/1  "Heading"

== system RoboBoatVU_2014_Athena/Sensors/Serial In/LIDAR Panda ==
  LIDAR Panda In : Inport
  ASCII Decode 2 : xpcseriallib/ASCII Decode   format=Color:%d\r\n  nvars=1  vartypes={'double'}
  FIFO ASCII read 1 : xpcseriallib/FIFO ASCII read   header={'Color:'}  term=[13 10]  hold=Hold last output if no new data  enable=off  maxsize=1024  outputtype=8 bit uint null terminated  sampletime=0.1
  LIDAR Panda Out : Outport
  wires:
  LIDAR Panda In/1 -> FIFO ASCII read 1/1
  FIFO ASCII read 1/1 -> ASCII Decode 2/1
  ASCII Decode 2/1 -> LIDAR Panda Out/1  "Buoy Color"

== system RoboBoatVU_2014_Athena/Sinks/actuators/analog output ==
  Compass Heading : Inport
  Control Signals : Inport  Port=2
  Analog output : speedgoatlib_IO102/Analog output  id=1  channels=[1,2,3,4]  range=2  ts=0.1  pciSlot=-1
  Ground : Ground
  Subsystem : Subsystem
  wires:
  Subsystem/1(Propulsion) -> Analog output/1
  Subsystem/2(Steering) -> Analog output/2
  Control Signals/1 -> Subsystem/2(Control Signals)
  Compass Heading/1 -> Subsystem/1(Compass Heading)
  Ground/1 -> Analog output/4, Analog output/3

== system RoboBoatVU_2014_Athena/Sinks/actuators/digital output ==
  Digital Out : Inport
  Digital output : speedgoatlib_IO102/Digital output  id=1  channels=[1,2,3,4,5,6,7,8]  ts=0.1  pciSlot=-1
  Ground : Ground
  Terminator : Terminator
  wires:
  Digital Out/1 -> Terminator/1
  Ground/1 -> Digital output/1, Digital output/2, Digital output/3, Digital output/4, Digital output/5, Digital output/6, Digital output/7, Digital output/8

== system RoboBoatVU_2014_Athena/Main FSM/Acoustic Location/Left Sample/Output Heirarchy ==
  Desired Heading : Inport
  Sensors : Inport  Port=2
  Annotated Image : Inport  Port=3
  Due Sample Start : Inport  Port=4
  Bus Creator : BusCreator  Inputs=3
  Bus Creator1 : BusCreator  Inputs=2
  Bus Creator2 : BusCreator  Inputs=3
  Bus Creator3 : BusCreator  Inputs=2
  Bus Creator4 : BusCreator  Inputs=2
  Finished : Constant  Value=0
  RPM Desired : Constant  Value=0
  Ready to Read : Constant  Value=0
  Uno Power : Constant  Value=0
  Outputs : Outport
  wires:
  RPM Desired/1 -> Bus Creator/1  "RPM"
  Bus Creator/1 -> Bus Creator1/1  "Control Signals"
  Bus Creator2/1 -> Bus Creator/3  "Arduino Signals"
  Uno Power/1 -> Bus Creator2/2  "Uno Power"
  Desired Heading/1 -> Bus Creator/2  "Desired Heading"
  Bus Creator1/1 -> Bus Creator4/1  "Outputs"
  Annotated Image/1 -> Bus Creator1/2  "Annotated Image"
  Sensors/1 -> Bus Creator4/2  "Sensors"
  Bus Creator4/1 -> Bus Creator3/1  "Output Signals"
  Ready to Read/1 -> Bus Creator2/1  "Ready to Read"
  Due Sample Start/1 -> Bus Creator2/3  "Due Sample Start"
  Bus Creator3/1 -> Outputs/1
  Finished/1 -> Bus Creator3/2  "Task Finished"

== system RoboBoatVU_2014_Athena/Main FSM/Acoustic Location/Left Turn/Output Heirarchy ==
  Desired Heading : Inport
  Sensors : Inport  Port=2
  Annotated Image : Inport  Port=3
  Bus Creator : BusCreator  Inputs=3
  Bus Creator1 : BusCreator  Inputs=2
  Bus Creator2 : BusCreator  Inputs=3
  Bus Creator3 : BusCreator  Inputs=2
  Bus Creator4 : BusCreator  Inputs=2
  Due Sample Start : Constant  Value=0
  Finished : Constant  Value=0
  RPM Desired : Constant  Value=0
  Ready to Read : Constant  Value=0
  Uno Power : Constant  Value=0
  Outputs : Outport
  wires:
  RPM Desired/1 -> Bus Creator/1  "RPM"
  Bus Creator/1 -> Bus Creator1/1  "Control Signals"
  Bus Creator2/1 -> Bus Creator/3  "Arduino Signals"
  Uno Power/1 -> Bus Creator2/2  "Uno Power"
  Desired Heading/1 -> Bus Creator/2  "Desired Heading"
  Bus Creator1/1 -> Bus Creator4/1  "Outputs"
  Annotated Image/1 -> Bus Creator1/2  "Annotated Image"
  Sensors/1 -> Bus Creator4/2  "Sensors"
  Bus Creator4/1 -> Bus Creator3/1  "Output Signals"
  Ready to Read/1 -> Bus Creator2/1  "Ready to Read"
  Due Sample Start/1 -> Bus Creator2/3  "Due Sample Start"
  Bus Creator3/1 -> Outputs/1
  Finished/1 -> Bus Creator3/2  "Task Finished"

== system RoboBoatVU_2014_Athena/Main FSM/Acoustic Location/Mid Sample/Output Heirarchy ==
  Desired Heading : Inport
  Sensors : Inport  Port=2
  Annotated Image : Inport  Port=3
  Due Sample Start : Inport  Port=4
  Bus Creator : BusCreator  Inputs=3
  Bus Creator1 : BusCreator  Inputs=2
  Bus Creator2 : BusCreator  Inputs=3
  Bus Creator3 : BusCreator  Inputs=2
  Bus Creator4 : BusCreator  Inputs=2
  Finished : Constant  Value=0
  RPM Desired : Constant  Value=0
  Ready to Read : Constant  Value=0
  Uno Power : Constant  Value=0
  Outputs : Outport
  wires:
  RPM Desired/1 -> Bus Creator/1  "RPM"
  Bus Creator/1 -> Bus Creator1/1  "Control Signals"
  Bus Creator2/1 -> Bus Creator/3  "Arduino Signals"
  Uno Power/1 -> Bus Creator2/2  "Uno Power"
  Desired Heading/1 -> Bus Creator/2  "Desired Heading"
  Bus Creator1/1 -> Bus Creator4/1  "Outputs"
  Annotated Image/1 -> Bus Creator1/2  "Annotated Image"
  Sensors/1 -> Bus Creator4/2  "Sensors"
  Bus Creator4/1 -> Bus Creator3/1  "Output Signals"
  Ready to Read/1 -> Bus Creator2/1  "Ready to Read"
  Due Sample Start/1 -> Bus Creator2/3  "Due Sample Start"
  Bus Creator3/1 -> Outputs/1
  Finished/1 -> Bus Creator3/2  "Task Finished"

== system RoboBoatVU_2014_Athena/Main FSM/Acoustic Location/Right Sample/Output Heirarchy1 ==
  Finished : Inport
  Desired Heading : Inport  Port=2
  Sensors : Inport  Port=3
  Annotated Image : Inport  Port=4
  Due Sample Start : Inport  Port=5
  Bus Creator : BusCreator  Inputs=3
  Bus Creator1 : BusCreator  Inputs=2
  Bus Creator2 : BusCreator  Inputs=3
  Bus Creator3 : BusCreator  Inputs=2
  Bus Creator4 : BusCreator  Inputs=2
  RPM Desired : Constant  Value=0
  Ready to Read : Constant  Value=0
  Uno Power : Constant  Value=0
  Outputs : Outport
  wires:
  RPM Desired/1 -> Bus Creator/1  "RPM"
  Bus Creator/1 -> Bus Creator1/1  "Control Signals"
  Bus Creator2/1 -> Bus Creator/3  "Arduino Signals"
  Uno Power/1 -> Bus Creator2/2  "Uno Power"
  Desired Heading/1 -> Bus Creator/2  "Desired Heading"
  Bus Creator1/1 -> Bus Creator4/1  "Outputs"
  Annotated Image/1 -> Bus Creator1/2  "Annotated Image"
  Sensors/1 -> Bus Creator4/2  "Sensors"
  Bus Creator4/1 -> Bus Creator3/1  "Output Signals"
  Ready to Read/1 -> Bus Creator2/1  "Ready to Read"
  Due Sample Start/1 -> Bus Creator2/3  "Due Sample Start"
  Bus Creator3/1 -> Outputs/1
  Finished/1 -> Bus Creator3/2  "Task Finished"

== system RoboBoatVU_2014_Athena/Main FSM/Acoustic Location/Right Turn/Output Heirarchy ==
  Desired Heading : Inport
  Sensors : Inport  Port=2
  Annotated Image : Inport  Port=3
  Bus Creator : BusCreator  Inputs=3
  Bus Creator1 : BusCreator  Inputs=2
  Bus Creator2 : BusCreator  Inputs=3
  Bus Creator3 : BusCreator  Inputs=2
  Bus Creator4 : BusCreator  Inputs=2
  Due Sample Start : Constant  Value=0
  Finished : Constant  Value=0
  RPM Desired : Constant  Value=0
  Ready to Read : Constant  Value=0
  Uno Power : Constant  Value=0
  Outputs : Outport
  wires:
  RPM Desired/1 -> Bus Creator/1  "RPM"
  Bus Creator/1 -> Bus Creator1/1  "Control Signals"
  Bus Creator2/1 -> Bus Creator/3  "Arduino Signals"
  Uno Power/1 -> Bus Creator2/2  "Uno Power"
  Desired Heading/1 -> Bus Creator/2  "Desired Heading"
  Bus Creator1/1 -> Bus Creator4/1  "Outputs"
  Annotated Image/1 -> Bus Creator1/2  "Annotated Image"
  Sensors/1 -> Bus Creator4/2  "Sensors"
  Bus Creator4/1 -> Bus Creator3/1  "Output Signals"
  Ready to Read/1 -> Bus Creator2/1  "Ready to Read"
  Due Sample Start/1 -> Bus Creator2/3  "Due Sample Start"
  Bus Creator3/1 -> Outputs/1
  Finished/1 -> Bus Creator3/2  "Task Finished"

== system RoboBoatVU_2014_Athena/Main FSM/Docking/Detection/Sort and Filter for Best Three ==
  BBox in : Inport
  Idx : Inport  Port=2
  First Three BBox : dspmtrx3/Submatrix  RowSpan=Range of rows  RowStartMode=First  RowStartIndex=1  RowEndMode=Index  RowEndIndex=3  ColSpan=Range of columns  ColStartMode=First  ColStartIndex=2  ColEndMode=Last  ColEndIndex=2
  Permute Matrix : dspmtrx3/Permute Matrix  mode=Rows  ZeroOneIdxMode=One-based  errmode=Clip index  checkDims=off
  Sort : dspstat3/Sort  otype=Index  dir=Ascending  sortAlg=Quick sort  accumDataTypeStr=Inherit: Same as product output  accumLastDataTypeStr=Inherit: Same as product output  roundingMode=Floor  overflowMode=off
  BBox out : Outport
  wires:
  First Three BBox/1 -> BBox out/1
  Permute Matrix/1 -> First Three BBox/1
  Sort/1 -> Permute Matrix/2
  Idx/1 -> Sort/1
  BBox in/1 -> Permute Matrix/1

== system RoboBoatVU_2014_Athena/Main FSM/Docking/Parameters/Templates ==
  Bus Creator : BusCreator  Inputs=3
  Circle : Constant  Value=|
      | [1	1	1	1	1	1	0	0	0	0	0	0	0	1	1	1	1	1	1
      | 1	1	1	1	0	0	0	0	0	0	0	0	0	0	0	1	1	1	1
      | 1	1	0	0	0	0	0	0	0	0	0	0	0	0	0	0	0	1	1
      | 1	1	0	0	0	0	0	0	0	0	0	0	0	0	0	0	0	1	1
      | 1	0	0	0	0	0	0	0	0	0	0	0	0	0	0	0	0	0	1
      | 1	0	0	0	0	0	0	0	0	0	0	0	0	0	0	0	0	0	1
      | 0	0	0	0	0	0	0	0	0	0	0	0	0	0	0	0	0	0	0
      | 0	0	0	0	0	0	0	0	0	0	0	0	0	0	0	0	0	0	0
      | 0	0	0	0	0	0	0	0	0	0	0	0	0	0	0	0	0	0	0
      | 0	0	0	0	0	0	0	0	0	0	0	0	0	0	0	0	0	0	0
      | 0	0	0	0	0	0	0	0	0	0	0	0	0	0	0	0	0	0	0
      | 0	0	0	0	0	0	0	0	0	0	0	0	0	0	0	0	0	0	0
      | 0	0	0	0	0	0	0	0	0	0	0	0	0	0	0	0	0	0	0
      | 1	0	0	0	0	0	0	0	0	0	0	0	0	0	0	0	0	0	1
      | 1	0	0	0	0	0	0	0	0	0	0	0	0	0	0	0	0	0	1
      | 1	1	0	0	0	0	0	0	0	0	0	0	0	0	0	0	0	1	1
      | 1	1	0	0	0	0	0	0	0	0	0	0	0	0	0	0	0	1	1
      | 1	1	1	1	0	0	0	0	0	0	0	0	0	0	0	1	1	1	1
      | 1	1	1	1	1	1	0	0	0	0	0	0	0	1	1	1	1	1	1]
  Cruciform : Constant  Value=|
      | [1	1	1	1	1	1	0	0	0	0	0	0	0	1	1	1	1	1	1
      | 1	1	1	1	1	1	0	0	0	0	0	0	0	1	1	1	1	1	1
      | 1	1	1	1	1	1	0	0	0	0	0	0	0	1	1	1	1	1	1
      | 1	1	1	1	1	1	0	0	0	0	0	0	0	1	1	1	1	1	1
      | 1	1	1	1	1	1	0	0	0	0	0	0	0	1	1	1	1	1	1
      | 1	1	1	1	1	1	0	0	0	0	0	0	0	1	1	1	1	1	1
      | 0	0	0	0	0	0	0	0	0	0	0	0	0	0	0	0	0	0	0
      | 0	0	0	0	0	0	0	0	0	0	0	0	0	0	0	0	0	0	0
      | 0	0	0	0	0	0	0	0	0	0	0	0	0	0	0	0	0	0	0
      | 0	0	0	0	0	0	0	0	0	0	0	0	0	0	0	0	0	0	0
      | 0	0	0	0	0	0	0	0	0	0	0	0	0	0	0	0	0	0	0
      | 0	0	0	0	0	0	0	0	0	0	0	0	0	0	0	0	0	0	0
      | 0	0	0	0	0	0	0	0	0	0	0	0	0	0	0	0	0	0	0
      | 1	1	1	1	1	1	0	0	0	0	0	0	0	1	1	1	1	1	1
      | 1	1	1	1	1	1	0	0	0	0	0	0	0	1	1	1	1	1	1
      | 1	1	1	1	1	1	0	0	0	0	0	0	0	1	1	1	1	1	1
      | 1	1	1	1	1	1	0	0	0	0	0	0	0	1	1	1	1	1	1
      | 1	1	1	1	1	1	0	0	0	0	0	0	0	1	1	1	1	1	1
      | 1	1	1	1	1	1	0	0	0	0	0	0	0	1	1	1	1	1	1]
  Triangle : Constant  Value=|
      | [1	1	1	1	1	1	1	1	1	0	1	1	1	1	1	1	1	1	1
      | 1	1	1	1	1	1	1	1	1	0	1	1	1	1	1	1	1	1	1
      | 1	1	1	1	1	1	1	1	0	0	0	1	1	1	1	1	1	1	1
      | 1	1	1	1	1	1	1	1	0	0	0	1	1	1	1	1	1	1	1
      | 1	1	1	1	1	1	1	0	0	0	0	0	1	1	1	1	1	1	1
      | 1	1	1	1	1	1	1	0	0	0	0	0	1	1	1	1	1	1	1
      | 1	1	1	1	1	1	0	0	0	0	0	0	0	1	1	1	1	1	1
      | 1	1	1	1	1	1	0	0	0	0	0	0	0	1	1	1	1	1	1
      | 1	1	1	1	1	0	0	0	0	0	0	0	0	0	1	1	1	1	1
      | 1	1	1	1	1	0	0	0	0	0	0	0	0	0	1	1	1	1	1
      | 1	1	1	1	0	0	0	0	0	0	0	0	0	0	0	1	1	1	1
      | 1	1	1	1	0	0	0	0	0	0	0	0	0	0	0	1	1	1	1
      | 1	1	1	0	0	0	0	0	0	0	0	0	0	0	0	0	1	1	1
      | 1	1	1	0	0	0	0	0	0	0	0	0	0	0	0	0	1	1	1
      | 1	1	0	0	0	0	0	0	0	0	0	0	0	0	0	0	0	1	1
      | 1	1	0	0	0	0	0	0	0	0	0	0	0	0	0	0	0	1	1
      | 1	0	0	0	0	0	0	0	0	0	0	0	0	0	0	0	0	0	1
      | 1	0	0	0	0	0	0	0	0	0	0	0	0	0	0	0	0	0	1
      | 0	0	0	0	0	0	0	0	0	0	0	0	0	0	0	0	0	0	0]
  Templates : Outport
  wires:
  Cruciform/1 -> Bus Creator/1  "Cruciform"
  Circle/1 -> Bus Creator/2  "Circle"
  Triangle/1 -> Bus Creator/3  "Triangle"
  Bus Creator/1 -> Templates/1

== system RoboBoatVU_2014_Athena/Main FSM/Docking/Recognition/Sort and Filter for Best One ==
  BBox in : Inport
  Idx : Inport  Port=2
  First BBox : dspmtrx3/Submatrix  RowSpan=One row  RowStartMode=First  RowStartIndex=1  RowEndMode=Index  RowEndIndex=1  ColSpan=All columns  ColStartMode=First  ColStartIndex=2  ColEndMode=Last  ColEndIndex=2
  Permute Matrix : dspmtrx3/Permute Matrix  mode=Rows  ZeroOneIdxMode=One-based  errmode=Clip index  checkDims=off
  Sort : dspstat3/Sort  otype=Index  dir=Ascending  sortAlg=Quick sort  accumDataTypeStr=Inherit: Same as product output  accumLastDataTypeStr=Inherit: Same as product output  roundingMode=Floor  overflowMode=off
  BBox out : Outport
  wires:
  First BBox/1 -> BBox out/1
  Permute Matrix/1 -> First BBox/1
  Sort/1 -> Permute Matrix/2
  Idx/1 -> Sort/1
  BBox in/1 -> Permute Matrix/1
